simulink model "PM_fnc1000_TestHarness_backup"  (R2022a)
settings: Solver=VariableStepAuto  StartTime=0.0  StopTime=10.0  RelTol=1e-3
values from neighbouring files (symbols this model uses):
  rate_ms = 10    [PM_fnc1000_tc01_iter01_testsignal_builder.m]    (also in PM_fnc21_tc01_iter01_testsignal_builder.m; PM_fnc22_tc01_iter01_testsignal_builder.m)
settings Model: Creator=306427  LastModifiedBy=306427

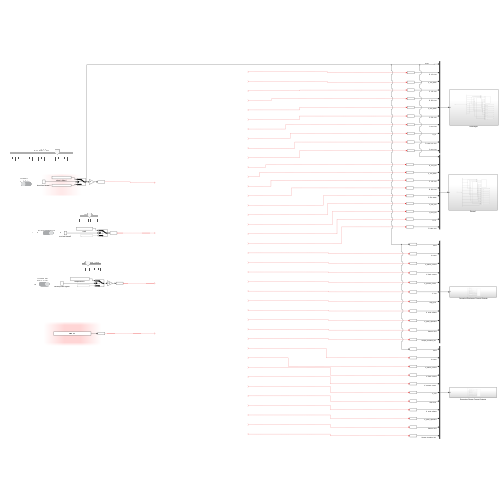
[thumbnail: Simulink's stored preview of the top-level diagram]
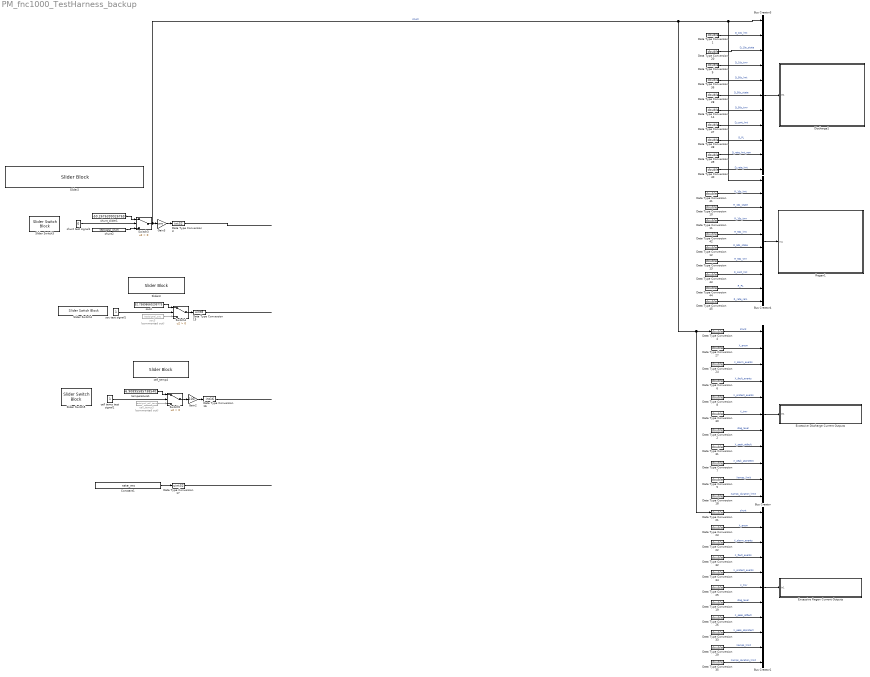
== system PM_fnc1000_TestHarness_backup ==
  Bus Creator : BusCreator  Inputs=11
  Bus Creator1 : BusCreator  Inputs=11
  Bus Creator3 : BusCreator  Inputs=11
  Bus Creator4 : BusCreator  Inputs=10
  Constant1 : Constant  Value=rate_ms
  Data Type Conversion{1..2,4..14,18..45} (41 alike) : DataTypeConversion  OutDataTypeStr=double  SaturateOnIntegerOverflow=off  RndMeth=Floor
  Data Type Conversion15 : DataTypeConversion  OutDataTypeStr=uint8  SaturateOnIntegerOverflow=off  RndMeth=Floor
  Data Type Conversion16 : DataTypeConversion  OutDataTypeStr=int16  SaturateOnIntegerOverflow=off  RndMeth=Floor
  Data Type Conversion17 : DataTypeConversion  OutDataTypeStr=uint32  SaturateOnIntegerOverflow=off  RndMeth=Floor
  Data Type Conversion3 : DataTypeConversion  OutDataTypeStr=int32  SaturateOnIntegerOverflow=off  RndMeth=Floor
  Discharge1 : Subsystem
  Excessive Discharge Current Outputs : Subsystem
  Excessive Regen Current Outputs : Subsystem
  Gain2 : Gain  Gain=100
  Gain3 : Gain  Gain=1000
  Regen1 : Subsystem
  Slider Switch3 : SliderSwitchBlock
      settings: Values={{'from wksp', 'slider'}, [0 1]}
  Slider Switch4 : SliderSwitchBlock
      settings: Values={{'soc from wksp', 'soc slider'}, [0 1]}
  Slider Switch5 : SliderSwitchBlock
      settings: Values={{'from wksp', 'slider'}, [0 1]}
  Slider2 : SliderBlock  ScaleMin=-1700  ScaleMax=+500
  Slider3 : SliderBlock
  Switch3 : Switch  Criteria=u2 > Threshold  SaturateOnIntegerOverflow=off  InputSameDT=off
  Switch4 : Switch  Criteria=u2 > Threshold  SaturateOnIntegerOverflow=off  InputSameDT=off
  Switch5 : Switch  Criteria=u2 > Threshold  SaturateOnIntegerOverflow=off  InputSameDT=off
  cell temp test signal1 : Constant
  cell_temp3 : FromWorkspace  Commented=on  VariableName=testsignal_cell_temp  OutDataTypeStr=double  SampleTime=[0, 1]
  cell_temp4 : SliderBlock  ScaleMin=-40  ScaleMax=70
  shunt test signal1 : Constant  Value=0
  shunt2 : FromWorkspace  VariableName=testsignal_shunt  OutDataTypeStr=double
  shunt_slider1 : Constant  Value=-50.26763990267659  OutDataTypeStr=double
  soc test signal1 : Constant
  soc3 : FromWorkspace  Commented=on  VariableName=testsignal_soc  OutDataTypeStr=double  SampleTime=[0, 1]
  soc4 : Constant  Value=52.75898660299775  OutDataTypeStr=double
  temperature1 : Constant  Value=-6.908955857385401  OutDataTypeStr=double
  wires:
  ? -> Data Type Conversion20/1
  cell_temp3/1 -> Switch5/3
  Data Type Conversion28/1 -> Bus Creator3/6  "D_50s_state"
  Data Type Conversion7/1 -> Bus Creator/9  "X_peak_atprotect"
  ? -> Data Type Conversion25/1
  Data Type Conversion35/1 -> Bus Creator1/11  "Xamps_duration_limit"
  Data Type Conversion26/1 -> Bus Creator1/8  "X_peak_atfault"
  shunt_slider1/1 -> Switch3/1
  ? -> Data Type Conversion11/1
  ? -> Data Type Conversion23/1
  Data Type Conversion19/1 -> Bus Creator1/7  "diag_level"
  Data Type Conversion31/1 -> Bus Creator/8  "X_peak_atfault"
  soc test signal1/1 -> Switch4/2
  ? -> Data Type Conversion1/1
  Data Type Conversion29/1 -> Bus Creator1/10  "Xamps_limit"
  ? -> Data Type Conversion5/1
  ? -> Data Type Conversion40/1
  Bus Creator/1 -> Excessive Discharge Current Outputs/1(In1)
  Data Type Conversion45/1 -> Bus Creator4/10  "R_rate_rem"
  Data Type Conversion39/1 -> Bus Creator3/10  "D_rate_lmt_rem"
  Data Type Conversion20/1 -> Bus Creator3/3  "D_10s_state"
  ? -> Data Type Conversion10/1
  Data Type Conversion22/1 -> Bus Creator1/3  "X_alarm_events"
  Data Type Conversion25/1 -> Bus Creator1/6  "X_tmr"
  ? -> Data Type Conversion19/1
  ? -> Data Type Conversion14/1
  ? -> Data Type Conversion38/1
  ? -> Data Type Conversion24/1
  ? -> Data Type Conversion30/1
  ? -> Data Type Conversion36/1
  Bus Creator4/1 -> Regen1/1(In1)
  Data Type Conversion24/1 -> Bus Creator/3  "X_alarm_events"
  Data Type Conversion36/1 -> Bus Creator3/5  "D_50s_lmt"
  ? -> Data Type Conversion42/1
  ? -> Data Type Conversion33/1
  ? -> Data Type Conversion32/1
  Data Type Conversion5/1 -> Bus Creator/10  "Xamps_limit"
  Switch4/1 -> Data Type Conversion15/1
  Data Type Conversion44/1 -> Bus Creator4/9  "R_PL"
  cell temp test signal1/1 -> Switch5/2
  Data Type Conversion14/1 -> Bus Creator3/7  "D_50s_tmr"
  Bus Creator1/1 -> Excessive Regen Current Outputs/1(In1)
  Data Type Conversion33/1 -> Bus Creator1/9  "X_peak_atprotect"
  ? -> Data Type Conversion12/1
  ? -> Data Type Conversion26/1
  ? -> Data Type Conversion22/1
  ? -> Data Type Conversion18/1
  Constant1/1 -> Data Type Conversion17/1
  ? -> Data Type Conversion35/1
  ? -> Data Type Conversion39/1
  ? -> Data Type Conversion6/1
  Data Type Conversion6/1 -> Bus Creator/4  "X_fault_events"
  ? -> Data Type Conversion9/1
  ? -> Data Type Conversion2/1
  Data Type Conversion37/1 -> Bus Creator3/8  "D_cont_lmt"
  ? -> Data Type Conversion7/1
  soc4/1 -> Switch4/1
  ? -> Data Type Conversion44/1
  temperature1/1 -> Switch5/1
  Data Type Conversion17/1 -> ?
  Data Type Conversion4/1 -> Bus Creator/1  "shunt"
  ? -> Data Type Conversion8/1
  Data Type Conversion42/1 -> Bus Creator4/5  "R_50s_lmt"
  Data Type Conversion30/1 -> Bus Creator/6  "X_tmr"
  ? -> Data Type Conversion28/1
  Data Type Conversion2/1 -> Bus Creator/7  "diag_level"
  ? -> Data Type Conversion41/1
  Data Type Conversion8/1 -> Bus Creator/5  "X_protect_events"
  shunt test signal1/1 -> Switch3/2
  ? -> Data Type Conversion34/1
  Switch5/1 -> Gain2/1
  Data Type Conversion41/1 -> Bus Creator4/2  "R_10s_lmt"
  Data Type Conversion32/1 -> Bus Creator1/4  "X_fault_events"
  ? -> Data Type Conversion37/1
  Data Type Conversion43/1 -> Bus Creator4/8  "R_cont_lmt"
  Data Type Conversion1/1 -> Bus Creator3/2  "D_10s_lmt"
  Data Type Conversion12/1 -> Bus Creator4/6  "R_50s_state"
  ? -> Data Type Conversion27/1
  Data Type Conversion27/1 -> Bus Creator/2  "X_enum"
  Gain3/1 -> Data Type Conversion3/1
  Gain2/1 -> Data Type Conversion16/1
  Data Type Conversion18/1 -> Bus Creator/11  "Xamps_duration_limit"
  Data Type Conversion9/1 -> Bus Creator3/4  "D_10s_tmr"
  soc3/1 -> Switch4/3
  Data Type Conversion13/1 -> Bus Creator4/7  "R_50s_tmr"
  ? -> Data Type Conversion43/1
  ? -> Data Type Conversion45/1
  Data Type Conversion11/1 -> Bus Creator4/4  "R_10s_tmr"
  Data Type Conversion34/1 -> Bus Creator1/5  "X_protect_events"
  Switch3/1 -> Bus Creator3/1, Bus Creator4/1, Data Type Conversion21/1, Data Type Conversion4/1, Gain3/1  "shunt"
  Data Type Conversion40/1 -> Bus Creator3/11  "D_rate_lmt"
  ? -> Data Type Conversion31/1
  ? -> Data Type Conversion29/1
  Data Type Conversion10/1 -> Bus Creator4/3  "R_10s_state"
  shunt2/1 -> Switch3/3
  Data Type Conversion15/1 -> ?
  Data Type Conversion23/1 -> Bus Creator1/2  "X_enum"
  ? -> Data Type Conversion13/1
  Data Type Conversion3/1 -> ?
  Data Type Conversion38/1 -> Bus Creator3/9  "D_PL"
  Bus Creator3/1 -> Discharge1/1(In1)
  Data Type Conversion21/1 -> Bus Creator1/1  "shunt"
  Data Type Conversion16/1 -> ?

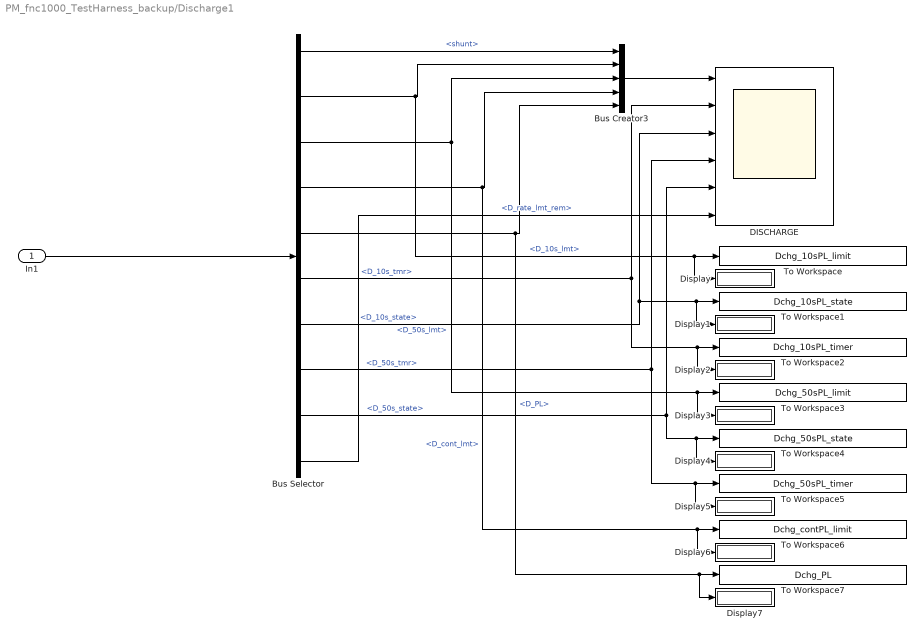
== system PM_fnc1000_TestHarness_backup/Discharge1 ==
  In1 : Inport
  Bus Creator3 : BusCreator  Inputs=5
  Bus Selector : BusSelector  OutputSignals=shunt,D_10s_lmt,D_50s_lmt,D_cont_lmt,D_PL,D_10s_tmr,D_10s_state,D_50s_tmr,D_50s_state,D_rate_lmt_rem
  DISCHARGE : Scope  NumInputPorts=6
  Display{,1..7} (8 alike) : Display
  To Workspace : ToWorkspace  VariableName=Dchg_10sPL_limit  SampleTime=-1
      settings: Save2DSignal=2-D array (concatenate along first dimension)
  To Workspace1 : ToWorkspace  VariableName=Dchg_10sPL_state  SampleTime=-1
      settings: Save2DSignal=2-D array (concatenate along first dimension)
  To Workspace2 : ToWorkspace  VariableName=Dchg_10sPL_timer  SampleTime=-1
      settings: Save2DSignal=2-D array (concatenate along first dimension)
  To Workspace3 : ToWorkspace  VariableName=Dchg_50sPL_limit  SampleTime=-1
      settings: Save2DSignal=2-D array (concatenate along first dimension)
  To Workspace4 : ToWorkspace  VariableName=Dchg_50sPL_state  SampleTime=-1
      settings: Save2DSignal=2-D array (concatenate along first dimension)
  To Workspace5 : ToWorkspace  VariableName=Dchg_50sPL_timer  SampleTime=-1
      settings: Save2DSignal=2-D array (concatenate along first dimension)
  To Workspace6 : ToWorkspace  VariableName=Dchg_contPL_limit  SampleTime=-1
      settings: Save2DSignal=2-D array (concatenate along first dimension)
  To Workspace7 : ToWorkspace  VariableName=Dchg_PL  SampleTime=-1
      settings: Save2DSignal=2-D array (concatenate along first dimension)
  wires:
  Bus Selector/5 -> To Workspace7/1, Display7/1, Bus Creator3/5  "<D_PL>"
  Bus Selector/9 -> DISCHARGE/5, To Workspace4/1, Display4/1  "<D_50s_state>"
  Bus Selector/2 -> To Workspace/1, Display/1, Bus Creator3/2  "<D_10s_lmt>"
  Bus Selector/4 -> To Workspace6/1, Display6/1, Bus Creator3/4  "<D_cont_lmt>"
  Bus Selector/7 -> To Workspace1/1, Display1/1, DISCHARGE/3  "<D_10s_state>"
  Bus Selector/6 -> To Workspace2/1, Display2/1, DISCHARGE/2  "<D_10s_tmr>"
  Bus Selector/10 -> DISCHARGE/6  "<D_rate_lmt_rem>"
  Bus Selector/8 -> To Workspace5/1, Display5/1, DISCHARGE/4  "<D_50s_tmr>"
  Bus Selector/3 -> To Workspace3/1, Display3/1, Bus Creator3/3  "<D_50s_lmt>"
  Bus Selector/1 -> Bus Creator3/1  "<shunt>"
  Bus Creator3/1 -> DISCHARGE/1
  In1/1 -> Bus Selector/1

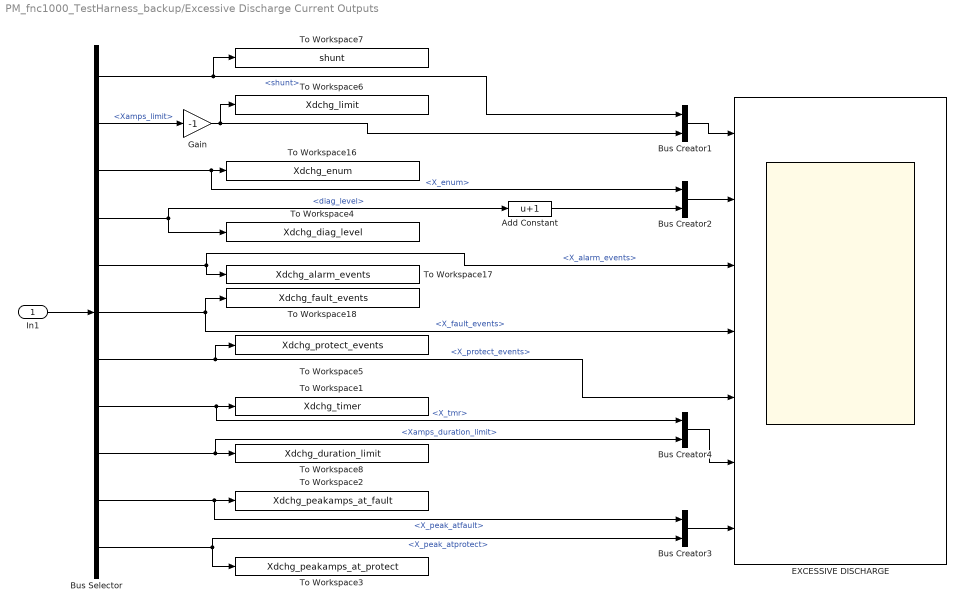
== system PM_fnc1000_TestHarness_backup/Excessive Discharge Current Outputs ==
  In1 : Inport
  Add Constant : Bias  Bias=1  SaturateOnIntegerOverflow=off
  Bus Creator{1..4} (4 alike) : BusCreator  Inputs=2
  Bus Selector : BusSelector  OutputSignals=shunt,Xamps_limit,X_enum,diag_level,X_alarm_events,X_fault_events,X_protect_events,X_tmr,Xamps_duration_limit,X_peak_atfault,X_peak_atprotect
  EXCESSIVE DISCHARGE : Scope  NumInputPorts=7
  Gain : Gain  Gain=-1
  To Workspace1 : ToWorkspace  VariableName=Xdchg_timer  SampleTime=-1
      settings: Save2DSignal=2-D array (concatenate along first dimension)
  To Workspace16 : ToWorkspace  VariableName=Xdchg_enum  SampleTime=-1
      settings: Save2DSignal=2-D array (concatenate along first dimension)
  To Workspace17 : ToWorkspace  VariableName=Xdchg_alarm_events  SampleTime=-1
      settings: Save2DSignal=2-D array (concatenate along first dimension)
  To Workspace18 : ToWorkspace  VariableName=Xdchg_fault_events  SampleTime=-1
      settings: Save2DSignal=2-D array (concatenate along first dimension)
  To Workspace2 : ToWorkspace  VariableName=Xdchg_peakamps_at_fault  SampleTime=-1
      settings: Save2DSignal=2-D array (concatenate along first dimension)
  To Workspace3 : ToWorkspace  VariableName=Xdchg_peakamps_at_protect  SampleTime=-1
      settings: Save2DSignal=2-D array (concatenate along first dimension)
  To Workspace4 : ToWorkspace  VariableName=Xdchg_diag_level  SampleTime=-1
      settings: Save2DSignal=2-D array (concatenate along first dimension)
  To Workspace5 : ToWorkspace  VariableName=Xdchg_protect_events  SampleTime=-1
      settings: Save2DSignal=2-D array (concatenate along first dimension)
  To Workspace6 : ToWorkspace  VariableName=Xdchg_limit  SampleTime=-1
      settings: Save2DSignal=2-D array (concatenate along first dimension)
  To Workspace7 : ToWorkspace  VariableName=shunt  SampleTime=-1
      settings: Save2DSignal=2-D array (concatenate along first dimension)
  To Workspace8 : ToWorkspace  VariableName=Xdchg_duration_limit  SampleTime=-1
      settings: Save2DSignal=2-D array (concatenate along first dimension)
  wires:
  In1/1 -> Bus Selector/1
  Bus Selector/3 -> Bus Creator2/1, To Workspace16/1  "<X_enum>"
  Gain/1 -> To Workspace6/1, Bus Creator1/2
  Bus Selector/5 -> EXCESSIVE DISCHARGE/3, To Workspace17/1  "<X_alarm_events>"
  Bus Creator1/1 -> EXCESSIVE DISCHARGE/1
  Bus Selector/1 -> To Workspace7/1, Bus Creator1/1  "<shunt>"
  Bus Selector/6 -> To Workspace18/1, EXCESSIVE DISCHARGE/4  "<X_fault_events>"
  Bus Selector/8 -> Bus Creator4/1, To Workspace1/1  "<X_tmr>"
  Bus Selector/10 -> To Workspace2/1, Bus Creator3/1  "<X_peak_atfault>"
  Bus Selector/2 -> Gain/1  "<Xamps_limit>"
  Bus Selector/4 -> Add Constant/1, To Workspace4/1  "<diag_level>"
  Bus Selector/11 -> To Workspace3/1, Bus Creator3/2  "<X_peak_atprotect>"
  Bus Selector/7 -> To Workspace5/1, EXCESSIVE DISCHARGE/5  "<X_protect_events>"
  Bus Creator2/1 -> EXCESSIVE DISCHARGE/2
  Bus Creator3/1 -> EXCESSIVE DISCHARGE/7
  Add Constant/1 -> Bus Creator2/2
  Bus Selector/9 -> To Workspace8/1, Bus Creator4/2  "<Xamps_duration_limit>"
  Bus Creator4/1 -> EXCESSIVE DISCHARGE/6

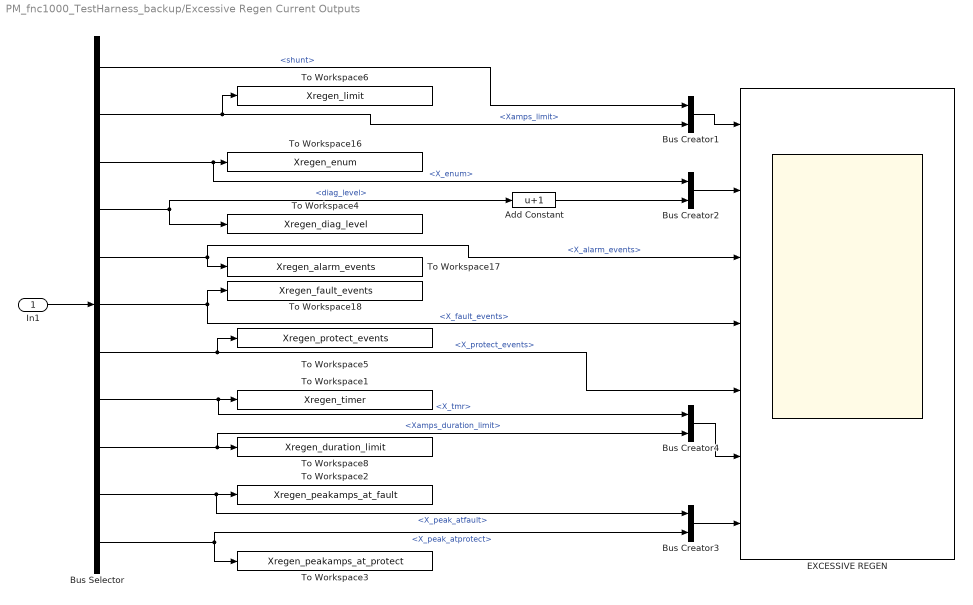
== system PM_fnc1000_TestHarness_backup/Excessive Regen Current Outputs ==
  In1 : Inport
  Add Constant : Bias  Bias=1  SaturateOnIntegerOverflow=off
  Bus Creator{1..4} (4 alike) : BusCreator  Inputs=2
  Bus Selector : BusSelector  OutputSignals=shunt,Xamps_limit,X_enum,diag_level,X_alarm_events,X_fault_events,X_protect_events,X_tmr,Xamps_duration_limit,X_peak_atfault,X_peak_atprotect
  EXCESSIVE REGEN : Scope  NumInputPorts=7
  To Workspace1 : ToWorkspace  VariableName=Xregen_timer  SampleTime=-1
      settings: Save2DSignal=2-D array (concatenate along first dimension)
  To Workspace16 : ToWorkspace  VariableName=Xregen_enum  SampleTime=-1
      settings: Save2DSignal=2-D array (concatenate along first dimension)
  To Workspace17 : ToWorkspace  VariableName=Xregen_alarm_events  SampleTime=-1
      settings: Save2DSignal=2-D array (concatenate along first dimension)
  To Workspace18 : ToWorkspace  VariableName=Xregen_fault_events  SampleTime=-1
      settings: Save2DSignal=2-D array (concatenate along first dimension)
  To Workspace2 : ToWorkspace  VariableName=Xregen_peakamps_at_fault  SampleTime=-1
      settings: Save2DSignal=2-D array (concatenate along first dimension)
  To Workspace3 : ToWorkspace  VariableName=Xregen_peakamps_at_protect  SampleTime=-1
      settings: Save2DSignal=2-D array (concatenate along first dimension)
  To Workspace4 : ToWorkspace  VariableName=Xregen_diag_level  SampleTime=-1
      settings: Save2DSignal=2-D array (concatenate along first dimension)
  To Workspace5 : ToWorkspace  VariableName=Xregen_protect_events  SampleTime=-1
      settings: Save2DSignal=2-D array (concatenate along first dimension)
  To Workspace6 : ToWorkspace  VariableName=Xregen_limit  SampleTime=-1
      settings: Save2DSignal=2-D array (concatenate along first dimension)
  To Workspace8 : ToWorkspace  VariableName=Xregen_duration_limit  SampleTime=-1
      settings: Save2DSignal=2-D array (concatenate along first dimension)
  wires:
  In1/1 -> Bus Selector/1
  Bus Selector/3 -> Bus Creator2/1, To Workspace16/1  "<X_enum>"
  Bus Selector/5 -> EXCESSIVE REGEN/3, To Workspace17/1  "<X_alarm_events>"
  Bus Creator1/1 -> EXCESSIVE REGEN/1
  Bus Selector/1 -> Bus Creator1/1  "<shunt>"
  Bus Selector/6 -> To Workspace18/1, EXCESSIVE REGEN/4  "<X_fault_events>"
  Bus Selector/8 -> Bus Creator4/1, To Workspace1/1  "<X_tmr>"
  Bus Selector/10 -> To Workspace2/1, Bus Creator3/1  "<X_peak_atfault>"
  Bus Selector/2 -> To Workspace6/1, Bus Creator1/2  "<Xamps_limit>"
  Bus Selector/4 -> Add Constant/1, To Workspace4/1  "<diag_level>"
  Bus Selector/11 -> To Workspace3/1, Bus Creator3/2  "<X_peak_atprotect>"
  Bus Selector/7 -> To Workspace5/1, EXCESSIVE REGEN/5  "<X_protect_events>"
  Bus Creator2/1 -> EXCESSIVE REGEN/2
  Bus Creator3/1 -> EXCESSIVE REGEN/7
  Add Constant/1 -> Bus Creator2/2
  Bus Selector/9 -> To Workspace8/1, Bus Creator4/2  "<Xamps_duration_limit>"
  Bus Creator4/1 -> EXCESSIVE REGEN/6

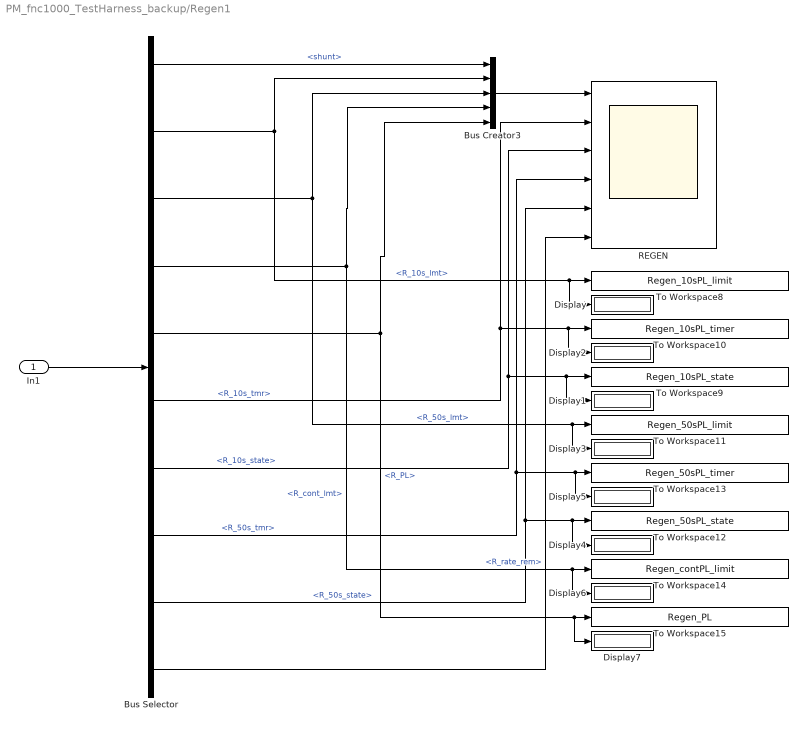
== system PM_fnc1000_TestHarness_backup/Regen1 ==
  In1 : Inport
  Bus Creator3 : BusCreator  Inputs=5
  Bus Selector : BusSelector  OutputSignals=shunt,R_10s_lmt,R_50s_lmt,R_cont_lmt,R_PL,R_10s_tmr,R_10s_state,R_50s_tmr,R_50s_state,R_rate_rem
  Display{,1..7} (8 alike) : Display
  REGEN : Scope  NumInputPorts=6
  To Workspace10 : ToWorkspace  VariableName=Regen_10sPL_timer  SampleTime=-1
      settings: Save2DSignal=2-D array (concatenate along first dimension)
  To Workspace11 : ToWorkspace  VariableName=Regen_50sPL_limit  SampleTime=-1
      settings: Save2DSignal=2-D array (concatenate along first dimension)
  To Workspace12 : ToWorkspace  VariableName=Regen_50sPL_state  SampleTime=-1
      settings: Save2DSignal=2-D array (concatenate along first dimension)
  To Workspace13 : ToWorkspace  VariableName=Regen_50sPL_timer  SampleTime=-1
      settings: Save2DSignal=2-D array (concatenate along first dimension)
  To Workspace14 : ToWorkspace  VariableName=Regen_contPL_limit  SampleTime=-1
      settings: Save2DSignal=2-D array (concatenate along first dimension)
  To Workspace15 : ToWorkspace  VariableName=Regen_PL  SampleTime=-1
      settings: Save2DSignal=2-D array (concatenate along first dimension)
  To Workspace8 : ToWorkspace  VariableName=Regen_10sPL_limit  SampleTime=-1
      settings: Save2DSignal=2-D array (concatenate along first dimension)
  To Workspace9 : ToWorkspace  VariableName=Regen_10sPL_state  SampleTime=-1
      settings: Save2DSignal=2-D array (concatenate along first dimension)
  wires:
  Bus Selector/5 -> To Workspace15/1, Display7/1, Bus Creator3/5  "<R_PL>"
  Bus Selector/2 -> To Workspace8/1, Display/1, Bus Creator3/2  "<R_10s_lmt>"
  Bus Selector/4 -> To Workspace14/1, Display6/1, Bus Creator3/4  "<R_cont_lmt>"
  Bus Selector/3 -> To Workspace11/1, Display3/1, Bus Creator3/3  "<R_50s_lmt>"
  Bus Selector/1 -> Bus Creator3/1  "<shunt>"
  Bus Creator3/1 -> REGEN/1
  In1/1 -> Bus Selector/1
  Bus Selector/10 -> REGEN/6  "<R_rate_rem>"
  Bus Selector/6 -> REGEN/2, Display2/1, To Workspace10/1  "<R_10s_tmr>"
  Bus Selector/7 -> REGEN/3, Display1/1, To Workspace9/1  "<R_10s_state>"
  Bus Selector/8 -> REGEN/4, Display5/1, To Workspace13/1  "<R_50s_tmr>"
  Bus Selector/9 -> REGEN/5, Display4/1, To Workspace12/1  "<R_50s_state>"
